simulink library "xrbsMath_r3"  (Simulink 5.0)
undefined symbols (not defined in the file or in its folder): num_width
libraries: xbsIndex_r3 x775, xrbsMath_r3 x16
(part 1 of 8)
settings Model: Creator=singhj  LastModifiedBy=singhj

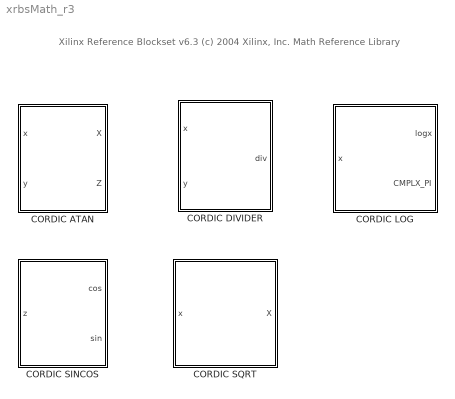
== system xrbsMath_r3 ==
  note: Xilinx Reference Blockset v6.3
      | (c) 2004  Xilinx, Inc.
      |
      | Math Reference Library
  CORDIC ATAN : Subsystem  mask{stages=8, pe_nbits=20, pe_binpt=15, pipeline_x=ones(1,8), prev_stages=8, pipeline=[1  1  1  1  1  1  1  1]}
      mask prompts: stages "Number of Processing Elements (integer value starting from 1)"; pe_nbits "X, Y Data Width"; pe_binpt "X, Y Binary Point Position"; pipeline_x "Latency for each Processing Element [1 0 0 1]"; prev_stages "Previous Number of Stages"; pipeline "Previous Pipeline Values"
      mask help: A parallel implementation, circular vectoring mode CORDIC processor for performing rectangular-to-polar conversion. The number of iteration stages (and resultant output accuracy) and the processor arithmetic precision are controlled by the mask customization.
      mask init:
      | [bg,fg] = xlcmap('XBlock',0);
      | iPos = get_param(gcb,'Position');
      | iWidth=iPos(3)-iPos(1); iHeight=iPos(4)-iPos(2);
      | iCx=iWidth/2;
      | iCy=iHeight/2;
      | [logoX, logoY] = xlogo(iPos);
      | sav_gcb=gcb;
      | stages = round(sum(abs(stages)));
      | if (stages == 0)
      | 	stages = prev_stages;
      | end
      | x = zeros(1,stages);
      | pipe_size = max(size(pipeline_x));
      | if pipe_size >= stages
      | 	x(1,1:stages) = pipeline_x(1,1:stages);
      | else
      | 	x(1,1:pipe_size) = pipeline_x(1,1:pipe_size);
      | end
      | 
      | if (stages ~=prev_stages)
      | 	pipeline=x;
      | 	cordic_pe = find_system(gcb, 'lookUnderMasks', 'all', 'FollowLinks','on','masktype', 'CORDIC parallel PE');
      |     
      |   a=find_system(cordic_pe{1}, 'lookUnderMasks', 'all', 'FollowLinks','on','masktype', 'CORDIC iteration PE');
      |   for i= 2:length(a)
      |     for j=1:3
      | 	  delete_line(cordic_pe{1}, ['CORDIC PE' int2str(i-1) '/' int2str(j)], ['CORDIC PE' int2str(i) '/' int2str(j)]);
      |     end
      |   end
      |     if length(a)>0,
      |       delete_line(cordic_pe{1}, 'x/1', 'CORDIC PE1/1');
      |       delete_line(cordic_pe{1}, 'y/1', 'CORDIC PE1/2');
      |       delete_line(cordic_pe{1}, 'z/1', 'CORDIC PE1/3');
      |       delete_line(cordic_pe{1}, ['CORDIC PE' int2str(length(a)) '/1'],'X/1');
      |       delete_line(cordic_pe{1}, ['CORDIC PE' int2str(length(a)) '/2'],'Terminator/1');
      |       delete_line(cordic_pe{1}, ['CORDIC PE' int2str(length(a)) '/3'],'Z/1');
      |     elseif length(a)==0
      |       temp_port=get_param([cordic_pe{1} '/x'],'porthandles');
      |       temp_line=get_param(temp_port.Outport,'line');
      |       if temp_line>=0  delete_line(temp_line); end
      |       temp_port=get_param([cordic_pe{1} '/y'],'porthandles');
      |       temp_line=get_param(temp_port.Outport,'line');
      |       if temp_line>=0  delete_line(temp_line); end
      |       temp_port=get_param([cordic_pe{1} '/z'],'porthandles');
      |       temp_line=get_param(temp_port.Outport,'line');
      |       if temp_line>=0  delete_line(temp_line); end
      |     end
      | 
      |     for i=2:length(a)
      |       delete_block(a{i});
      |     end
      |     for i=2:stages,
      |         add_block([cordic_pe{1} '/CORDIC PE1'], [cordic_pe{1} '/CORDIC PE' int2str(i)], 'ii', int2str(i-1),'pe_nbits', 'pe_nbits','pe_binpt', 'pe_binpt','pipeline',['pipeline(1,' int2str(i) ')'],'position',[150+(i-1)*125, 70, 205+(i-1)*125, 130]);
      |     end
      | 
      |     for i= 2:stages,
      |       for j=1:3
      | 		add_line(cordic_pe{1}, ['CORDIC PE' int2str(i-1) '/' int2str(j)], ['CORDIC PE' int2str(i) '/' int2str(j)], 'autorouting', 'on');
      |       end
      |     end
      | 
      |     if stages==0
      |       add_line(cordic_pe{1}, 'x/1', 'X/1', 'autorouting', 'on');
      |       add_line(cordic_pe{1}, 'y/1', 'Terminator/1', 'autorouting', 'on');
      |       add_line(cordic_pe{1}, 'z/1', 'Z/1', 'autorouting', 'on');
      |     elseif stages>0
      |       add_line(cordic_pe{1}, 'x/1', 'CORDIC PE1/1', 'autorouting', 'on');
      |       add_line(cordic_pe{1}, 'y/1', 'CORDIC PE1/2', 'autorouting', 'on');
      |       add_line(cordic_pe{1}, 'z/1', 'CORDIC PE1/3', 'autorouting', 'on');
      | 
      |       set_param([cordic_pe{1} '/' 'X'], 'Position', [150+stages*125, 72, 180+stages*125, 86]);
      |       set_param([cordic_pe{1} '/' 'Terminator'], 'Position', [210+stages*125, 92, 225+stages*125, 108]);
      |       set_param([cordic_pe{1} '/' 'Z'], 'Position', [240+stages*125, 113, 270+stages*125, 127]);
      | 
      |       add_line(cordic_pe{1}, ['CORDIC PE' int2str(stages) '/1'], 'X/1', 'autorouting', 'on');
      |       add_line(cordic_pe{1}, ['CORDIC PE' int2str(stages) '/2'], 'Terminator/1', 'autorouting', 'on');
      |       add_line(cordic_pe{1}, ['CORDIC PE' int2str(stages) '/3'],'Z/1', 'autorouting', 'on');
      | 
      |       % force a "compile" of the constituent constant blocks to
      |       % workaround a data propagation problem
      |       find_system(cordic_pe{1}, 'lookUnderMasks', 'all', 'FollowLinks', 'on', 'MaskType','Xilinx Constant Block');
      |   end
      | 	set_param(sav_gcb, 'prev_stages', int2str(stages));
      | 	set_param(sav_gcb, 'pipeline', [ '[' int2str(x) ']']);
      | else
      | 	if (sum(pipeline~=x))
      | 		set_param(gcb, 'pipeline', [ '[' int2str(x) ']']);
      | 	end
      | end
      | str = sprintf('-%d',sum(x) + 3);
      settings: CopyFcn=set_param(gcb, 'MaskSelfModifiable', 'on', 'LinkStatus', 'none');
      mask Help: web(xlhtmldoclink('CORDIC ATAN'));
      mask Display:
      | patch([0 iWidth iWidth 0],[0 0 iHeight iHeight] , bg);
      | patch(logoX,logoY , fg);
      | text(iCx-6,iCy,'z');
      | text(iCx,iCy+4,str);
      | port_label('input',1,'x');
      | port_label('input',2,'y');
      | port_label('output',1,'mag');
      | port_label('output',2,'atan');
      | plot([0 0 iWidth iWidth 0], [0 iHeight iHeight 0 0]);
  CORDIC DIVIDER : Subsystem  mask(CORDIC Based Divider){stages=11, num_width=16, num_binpt=11, pipeline_x=ones(1,11), prev_stages=11, pipeline=[1  1  1  1  1  1  1  1  1  1  1], prev_bits=15}
      mask prompts: stages "Number of Processing Elements (integer value starting from 1)"; num_width "X, Y, Data Width"; num_binpt "X,Y Binary Point Position"; pipeline_x "Latency for each Processing Element [1 0 0 1]"; prev_stages "Previous Number of Stages"; pipeline "Previous Pipeline Value"; prev_bits "Previous Number of Bits"
      mask help: This design implements a divider circuit using a fully parallel CORDIC (COordinate Rotation DIgital Computer) algorithm in linear vectoring mode with pre and post compensation. Using pre and post compensation techniques, this design can compute any arbitrary ratio y/x.
      mask init:
      | [bg,fg] = xlcmap('XBlock',0);
      | iPos = get_param(gcb,'Position');
      | iWidth=iPos(3)-iPos(1); iHeight=iPos(4)-iPos(2);
      | iCx=iWidth/2;
      | iCy=iHeight/2;
      | [logoX, logoY] = xlogo(iPos);
      | sav_gcb=gcb;
      | stages = round(sum(abs(stages)));
      | if (stages == 0)
      | 	stages = prev_stages;
      | end
      | x = zeros(1,stages);
      | pipe_size = max(size(pipeline_x));
      | if pipe_size >= stages
      | 	x(1,1:stages) = pipeline_x(1,1:stages);
      | else
      | 	x(1,1:pipe_size) = pipeline_x(1,1:pipe_size);
      | end
      | 
      | num_width = round(sum(abs(num_width)));
      | if (num_width < 2)
      | 	num_width = prev_bits;
      | end
      | 
      | if ((num_width-1) ~=prev_bits)
      |     % Draw the Normalization X Stage
      |     norm_x = find_system(sav_gcb, 'lookUnderMasks', 'all', 'FollowLinks','on','masktype', 'Normalize X');
      | 	a=find_system(norm_x{1}, 'lookUnderMasks', 'all', 'FollowLinks','on','masktype', 'Normalize Shift Stage');
      | 	for i= 2:length(a)
      | 		for j=1:3
      | 		    delete_line(norm_x{1}, ['Shift' int2str(i-1) '/' int2str(j)], ['Shift' int2str(i) '/' int2str(j)]);
      | 		end
      | 	end
      | 	delete_line(norm_x{1}, ['Shift' int2str(length(a)) '/1'],'norm/1');
      | 	delete_line(norm_x{1}, ['Shift' int2str(length(a)) '/2'],'shift/1');
      | 	delete_line(norm_x{1}, ['Shift' int2str(length(a)) '/3'],'Terminator1/1');
      | 	
      | 	for i=2:length(a)
      |       delete_block(a{i});
      | 	end
      | 	for i=2:(num_width-1),
      |         add_block([norm_x{1} '/Shift1'], [norm_x{1} '/Shift' int2str(i)],'position',[150+(i-1)*125, 70, 205+(i-1)*125, 130]);
      | 	end
      |     set_param([norm_x{1} '/' 'norm'], 'Position', [150+i*125, 72, 180+i*125, 86]);
      |     set_param([norm_x{1} '/' 'shift'], 'Position', [210+i*125, 92, 225+i*125, 108]);
      |     set_param([norm_x{1} '/' 'Terminator1'], 'Position', [240+i*125, 113, 270+i*125, 127]);
      |     for i= 2:(num_width-1)
      | 		for j=1:3
      | 		    add_line(norm_x{1}, ['Shift' int2str(i-1) '/' int2str(j)], ['Shift' int2str(i) '/' int2str(j)]);
      | 		end
      | 	end
      |     add_line(norm_x{1}, ['Shift' int2str((num_width-1)) '/1'],'norm/1');
      | 	add_line(norm_x{1}, ['Shift' int2str((num_width-1)) '/2'],'shift/1');
      | 	add_line(norm_x{1}, ['Shift' int2str((num_width-1)) '/3'],'Terminator1/1');
      |     
      |     % Draw the Normalization Y Stage
      |     norm_y = find_system(sav_gcb, 'lookUnderMasks', 'all', 'FollowLinks','on','masktype', 'Normalize Y');
      | 	a=find_system(norm_y{1}, 'lookUnderMasks', 'all', 'FollowLinks','on','masktype', 'Normalize Shift Stage');
      | 	for i= 2:length(a)
      | 		for j=1:3
      | 		    delete_line(norm_y{1}, ['Shift' int2str(i-1) '/' int2str(j)], ['Shift' int2str(i) '/' int2str(j)]);
      | 		end
      | 	end
      | 	delete_line(norm_y{1}, ['Shift' int2str(length(a)) '/1'],'norm/1');
      | 	delete_line(norm_y{1}, ['Shift' int2str(length(a)) '/2'],'shift/1');
      | 	delete_line(norm_y{1}, ['Shift' int2str(length(a)) '/3'],'Terminator1/1');
      | 	
      | 	for i=2:length(a)
      |       delete_block(a{i});
      | 	end
      | 	for i=2:(num_width-1)
      |         add_block([norm_y{1} '/Shift1'], [norm_y{1} '/Shift' int2str(i)],'position',[150+(i-1)*125, 70, 205+(i-1)*125, 130]);
      | 	end
      |     set_param([norm_y{1} '/' 'norm'], 'Position', [150+i*125, 72, 180+i*125, 86]);
      |     set_param([norm_y{1} '/' 'shift'], 'Position', [210+i*125, 92, 225+i*125, 108]);
      |     set_param([norm_y{1} '/' 'Terminator1'], 'Position', [240+i*125, 113, 270+i*125, 127]);
      |     for i= 2:(num_width-1)
      | 		for j=1:3
      | 		    add_line(norm_y{1}, ['Shift' int2str(i-1) '/' int2str(j)], ['Shift' int2str(i) '/' int2str(j)]);
      | 		end
      | 	end
      |     add_line(norm_y{1}, ['Shift' int2str((num_width-1)) '/1'],'norm/1');
      | 	add_line(norm_y{1}, ['Shift' int2str((num_width-1)) '/2'],'shift/1');
      | 	add_line(norm_y{1}, ['Shift' int2str((num_width-1)) '/3'],'Terminator1/1');
      | 	find_system(sav_gcb, 'lookUnderMasks', 'all', 'FollowLinks', 'on', 'MaskType','Xilinx Multiplexer Block');
      | 	set_param(sav_gcb, 'prev_bits',int2str((num_width-1)));
      | end
      | if (stages ~=prev_stages)
      | 	pipeline=x;
      |     iterative_divider = find_system(sav_gcb, 'lookUnderMasks', 'all', 'FollowLinks','on','masktype', 'CORDIC Iterative Divider');
      |   a=find_system(iterative_divider{1}, 'lookUnderMasks', 'all', 'FollowLinks','on','masktype', 'CORDIC iteration Divider');
      |   for i= 2:length(a)
      |     for j=1:3
      | 	  delete_line(iterative_divider{1}, ['CORDIC PE' int2str(i-1) '/' int2str(j)], ['CORDIC PE' int2str(i) '/' int2str(j)]);
      |     end
      |   end
      |   delete_line(iterative_divider{1}, ['CORDIC PE' int2str(length(a)) '/1'],'Terminator1/1');
      |   delete_line(iterative_divider{1}, ['CORDIC PE' int2str(length(a)) '/2'],'Terminator2/1');
      |   delete_line(iterative_divider{1}, ['CORDIC PE' int2str(length(a)) '/3'],'Z/1');
      |   for i=2:length(a)
      |      delete_block(a{i});
      |   end
      |   for i=2:stages,
      |       add_block([iterative_divider{1} '/CORDIC PE1'], [iterative_divider{1} '/CORDIC PE' int2str(i)], 'ii', int2str(i-1),'pipeline',['pipeline(1,' int2str(i) ')'],'position',[150+(i-1)*125, 70, 205+(i-1)*125, 130]);
      |   end
      |   for i= 2:stages,
      |      for j=1:3
      | 	     add_line(iterative_divider{1}, ['CORDIC PE' int2str(i-1) '/' int2str(j)], ['CORDIC PE' int2str(i) '/' int2str(j)], 'autorouting', 'on');
      |      end
      |   end
      |   set_param([iterative_divider{1} '/' 'Terminator1'], 'Position', [150+stages*125, 72, 180+stages*125, 86]);
      |   set_param([iterative_divider{1} '/' 'Terminator2'], 'Position', [210+stages*125, 92, 225+stages*125, 108]);
      |   set_param([iterative_divider{1} '/' 'Z'], 'Position', [240+stages*125, 113, 270+stages*125, 127]);
      | 
      |   add_line(iterative_divider{1}, ['CORDIC PE' int2str(stages) '/1'], 'Terminator1/1', 'autorouting', 'on');
      |   add_line(iterative_divider{1}, ['CORDIC PE' int2str(stages) '/2'], 'Terminator2/1', 'autorouting', 'on');
      |   add_line(iterative_divider{1}, ['CORDIC PE' int2str(stages) '/3'],'Z/1', 'autorouting', 'on');
      |    % force a "compile" of the constituent constant blocks to
      |    % workaround a data propagation problem
      |    find_system(iterative_divider{1}, 'lookUnderMasks', 'all', 'FollowLinks', 'on', 'MaskType','Xilinx Constant Block');
      |    set_param(sav_gcb, 'prev_stages', int2str(stages));
      |    set_param(sav_gcb, 'pipeline', [ '[' int2str(x) ']']);
      | else
      | 	if (sum(pipeline~=x))
      | 		set_param(sav_gcb, 'pipeline', [ '[' int2str(x) ']']);
      | 	end
      | end
      | 
      | str = sprintf('-%d',sum(x) + num_width + 4);
      settings: CopyFcn=set_param(gcb, 'MaskSelfModifiable', 'on', 'LinkStatus', 'none');
      mask Help: web(xlhtmldoclink('CORDIC DIVIDER'));
      mask Display:
      | patch([0 iWidth iWidth 0],[0 0 iHeight iHeight] , bg);
      | patch(logoX,logoY , fg);
      | text(iCx-6,iCy,'z');
      | text(iCx,iCy+4,str);
      | port_label('input',1,'x');
      | port_label('input',2,'y');
      | port_label('output',1,'y/x');
      | plot([0 0 iWidth iWidth 0], [0 iHeight iHeight 0 0]);
  CORDIC LOG : Subsystem  mask{stages=8, pe_nbits=8, pe_binpt=4, pipeline=ones(1,8), norm_nbits=0, norm_binpt=0}
      mask prompts: stages "Number of Processing Elements (integer value starting from 1)"; pe_nbits "Input Data Width"; pe_binpt "Input Binary Point Position"; pipeline "Latency for each Processing Element [1 0 0 1]"; norm_nbits "Normalized Data Width"; norm_binpt "Normalized Binary Point Position"
      mask help: A parallel implementation, hyperbolic vectoring mode CORDIC processor for calculating natural log of input x. The number of iteration stages (and resultant output accuracy) and the processor arithmetic precision are controlled by the mask customization.
      mask init:
      | [bg,fg] = xlcmap('XBlock',0);
      | iPos = get_param(gcb,'Position');
      | iWidth=iPos(3)-iPos(1); iHeight=iPos(4)-iPos(2);
      | iCx=iWidth/2;
      | iCy=iHeight/2;
      | [logoX, logoY] = xlogo(iPos);
      | 
      | if(length(pipeline)>stages)
      | 	x = sum(pipeline(1,1:stages));
      | else
      | 	x = sum(pipeline);
      | end
      | 
      | str = sprintf('-%d',2+pe_nbits-1+x+1);
      settings: CopyFcn=set_param(gcb, 'MaskSelfModifiable', 'on', 'LinkStatus', 'none');
      mask Help: web(xlhtmldoclink('CORDIC LOG'));
      mask Display:
      | patch([0 iWidth iWidth 0],[0 0 iHeight iHeight] , bg);
      | patch(logoX,logoY , fg);
      | text(iCx-6,iCy,'z');
      | text(iCx,iCy+4,str);
      | port_label('input',1,'x');
      | port_label('output',1,'log x');
      | port_label('output',2,'CMPLX_PI');
      | plot([0 0 iWidth iWidth 0], [0 iHeight iHeight 0 0]);
  CORDIC SINCOS : Subsystem  mask(CORDIC based Sine and Cosine function){stages=8, pe_nbits=16, pe_binpt=13, pipeline_x=ones(1,8), prev_stages=8, pipeline=[1  1  1  1  1  1  1  1]}
      mask prompts: stages "Number of Processing Elements (integer value starting from 1)"; pe_nbits "Input Data Width"; pe_binpt "Input Binary Point Position"; pipeline_x "Latency for each Processing Element [1 0 0 1]"; prev_stages "Previous Number of Stages"; pipeline "Previous Pipeline Values"
      mask help: A parallel implementation, circular rotation mode CORDIC processor for calculating Sine and Cosine of input angle z. The number of iteration stages (and resultant output accuracy) and the processor arithmetic precision are controlled by the mask customization.
      mask init:
      | [bg,fg] = xlcmap('XBlock',0);
      | iPos = get_param(gcb,'Position');
      | iWidth=iPos(3)-iPos(1); iHeight=iPos(4)-iPos(2);
      | iCx=iWidth/2;
      | iCy=iHeight/2;
      | [logoX, logoY] = xlogo(iPos);
      | sav_gcb=gcb;
      | stages = round(sum(abs(stages)));
      | if (stages == 0)
      | 	stages = prev_stages;
      | end
      | x = zeros(1,stages);
      | pipe_size = max(size(pipeline_x));
      | if pipe_size >= stages
      | 	x(1,1:stages) = pipeline_x(1,1:stages);
      | else
      | 	x(1,1:pipe_size) = pipeline_x(1,1:pipe_size);
      | end
      | 
      | if (stages ~=prev_stages)
      | 	pipeline=x;
      | 	cordic_pe = find_system(gcb, 'lookUnderMasks', 'all', 'FollowLinks','on','masktype', 'CORDIC parallel PE');
      |     
      |   a=find_system(cordic_pe{1}, 'lookUnderMasks', 'all', 'FollowLinks','on','masktype', 'CORDIC iteration PE');
      |   for i= 2:length(a)
      |     for j=1:3
      | 	  delete_line(cordic_pe{1}, ['CORDIC PE' int2str(i-1) '/' int2str(j)], ['CORDIC PE' int2str(i) '/' int2str(j)]);
      |     end
      |   end
      |     if length(a)>0,
      |       delete_line(cordic_pe{1}, 'x/1', 'CORDIC PE1/1');
      |       delete_line(cordic_pe{1}, 'y/1', 'CORDIC PE1/2');
      |       delete_line(cordic_pe{1}, 'z/1', 'CORDIC PE1/3');
      |       delete_line(cordic_pe{1}, ['CORDIC PE' int2str(length(a)) '/1'],'X/1');
      |       delete_line(cordic_pe{1}, ['CORDIC PE' int2str(length(a)) '/2'],'Y/1');
      |       delete_line(cordic_pe{1}, ['CORDIC PE' int2str(length(a)) '/3'],'Terminator/1');
      |     elseif length(a)==0
      |       temp_port=get_param([cordic_pe{1} '/x'],'porthandles');
      |       temp_line=get_param(temp_port.Outport,'line');
      |       if temp_line>=0  delete_line(temp_line); end
      |       temp_port=get_param([cordic_pe{1} '/y'],'porthandles');
      |       temp_line=get_param(temp_port.Outport,'line');
      |       if temp_line>=0  delete_line(temp_line); end
      |       temp_port=get_param([cordic_pe{1} '/z'],'porthandles');
      |       temp_line=get_param(temp_port.Outport,'line');
      |       if temp_line>=0  delete_line(temp_line); end
      |     end
      | 
      |     for i=2:length(a)
      |       delete_block(a{i});
      |     end
      |     for i=2:stages,
      |         add_block([cordic_pe{1} '/CORDIC PE1'], [cordic_pe{1} '/CORDIC PE' int2str(i)], 'ii', int2str(i-1),'pe_nbits', 'pe_nbits','pe_binpt', 'pe_binpt','pipeline',['pipeline(1,' int2str(i) ')'],'position',[150+(i-1)*125, 70, 205+(i-1)*125, 130]);
      |     end
      | 
      |     for i= 2:stages,
      |       for j=1:3
      | 		add_line(cordic_pe{1}, ['CORDIC PE' int2str(i-1) '/' int2str(j)], ['CORDIC PE' int2str(i) '/' int2str(j)], 'autorouting', 'on');
      |       end
      |     end
      | 
      |     if stages==0
      |       add_line(cordic_pe{1}, 'x/1', 'X/1', 'autorouting', 'on');
      |       add_line(cordic_pe{1}, 'y/1', 'Terminator/1', 'autorouting', 'on');
      |       add_line(cordic_pe{1}, 'z/1', 'Z/1', 'autorouting', 'on');
      |     elseif stages>0
      |       add_line(cordic_pe{1}, 'x/1', 'CORDIC PE1/1', 'autorouting', 'on');
      |       add_line(cordic_pe{1}, 'y/1', 'CORDIC PE1/2', 'autorouting', 'on');
      |       add_line(cordic_pe{1}, 'z/1', 'CORDIC PE1/3', 'autorouting', 'on');
      | 
      |       set_param([cordic_pe{1} '/' 'X'], 'Position', [150+stages*125, 72, 180+stages*125, 86]);
      |       set_param([cordic_pe{1} '/' 'Y'], 'Position', [210+stages*125, 92, 225+stages*125, 108]);
      |       set_param([cordic_pe{1} '/' 'Terminator'], 'Position', [240+stages*125, 113, 270+stages*125, 127]);
      | 
      |       add_line(cordic_pe{1}, ['CORDIC PE' int2str(stages) '/1'], 'X/1', 'autorouting', 'on');
      |       add_line(cordic_pe{1}, ['CORDIC PE' int2str(stages) '/2'], 'Y/1', 'autorouting', 'on');
      |       add_line(cordic_pe{1}, ['CORDIC PE' int2str(stages) '/3'],'Terminator/1', 'autorouting', 'on');
      | 
      |       % force a "compile" of the constituent constant blocks to
      |       % workaround a data propagation problem
      |       find_system(cordic_pe{1}, 'lookUnderMasks', 'all', 'FollowLinks', 'on', 'MaskType','Xilinx Constant Block');
      |   end
      | 	set_param(sav_gcb, 'prev_stages', int2str(stages));
      | 	set_param(sav_gcb, 'pipeline', [ '[' int2str(x) ']']);
      | else
      | 	if (sum(pipeline~=x))
      | 		set_param(gcb, 'pipeline', [ '[' int2str(x) ']']);
      | 	end
      | end
      | str = sprintf('-%d',sum(x) + 3);
      settings: CopyFcn=set_param(gcb, 'MaskSelfModifiable', 'on', 'LinkStatus', 'none');
      mask Help: web(xlhtmldoclink('CORDIC SINCOS'));
      mask Display:
      | patch([0 iWidth iWidth 0],[0 0 iHeight iHeight] , bg);
      | patch(logoX,logoY , fg);
      | text(iCx-6,iCy,'z');
      | text(iCx,iCy+4,str);
      | port_label('input',1,'z');
      | port_label('output',1,'cos');
      | port_label('output',2,'sin');
      | plot([0 0 iWidth iWidth 0], [0 iHeight iHeight 0 0]);
  CORDIC SQRT : Subsystem  mask{stages=12, pe_nbits=12, pe_binpt=6, pipeline=ones(1,12), norm_nbits=0, norm_binpt=0}
      mask prompts: stages "Number of Processing Elements (integer value starting from 1)"; pe_nbits "Input Data Width"; pe_binpt "Input Binary Point Position"; pipeline "Latency for each Processing Element [1 0 0 1]"; norm_nbits "Normalized Data Width"; norm_binpt "Normalized Binary Point"
      mask help: A parallel implementation, hyperbolic vectoring mode CORDIC processor for calculating square root of input x. The number of iteration stages (and resultant output accuracy) and the processor arithmetic precision are controlled by the mask customization.
      mask init:
      | [bg,fg] = xlcmap('XBlock',0);
      | iPos = get_param(gcb,'Position');
      | iWidth=iPos(3)-iPos(1); iHeight=iPos(4)-iPos(2);
      | iCx=iWidth/2;
      | iCy=iHeight/2;
      | [logoX, logoY] = xlogo(iPos);
      | %Normalized Data Width
      | norm_nbits = pe_binpt + (pe_nbits-pe_binpt) + mod(pe_nbits-pe_binpt-1,2);
      | norm_binpt = norm_nbits-1;
      | 
      | if(length(pipeline)>stages)
      | 	x = sum(pipeline(1,1:stages));
      | else
      | 	x = sum(pipeline);
      | end
      | 
      | str = sprintf('-%d',2+norm_binpt+1+x + 4);
      settings: CopyFcn=set_param(gcb, 'MaskSelfModifiable', 'on', 'LinkStatus', 'none');
      mask Help: web(xlhtmldoclink('CORDIC SQRT'));
      mask Display:
      | patch([0 iWidth iWidth 0],[0 0 iHeight iHeight] , bg);
      | patch(logoX,logoY , fg);
      | text(iCx-6,iCy,'z');
      | text(iCx,iCy+4,str);
      | port_label('input',1,'x');
      | port_label('output',1,'sqrt x');
      | plot([0 0 iWidth iWidth 0], [0 iHeight iHeight 0 0]);

== system xrbsMath_r3/CORDIC ATAN ==
  note: The CORDIC algorithm is implemented in 3 steps.
      |
      | Step 1: Coarse Angle Rotation.  The algorithm converges only for angles between -pi/2 and pi/2, so if x < zero, the input vector is reflected
      | to the 1st or 3rd quadrant by making the x-coordinate non-negative.
      |
      | Step 2: Fine Angle Rotation.  For rectangular-to-polar conversion, the resulting vector is rotated through progressively smaller angles, such that y goes
      | to zero. In the i-th stage, the angular rotation is by either +/- atan(1/2^i), depending on whether or not its input y is less than or greater than zero.
      |
      | Step 3: Angle Correction. If there was a reflection applied in Step 1, this step applies the appropriate angle correction by subtracting it from +/- pi.
  x : Inport
  y : Inport  Port=2
  CORDIC  Pipe Balance : xbsIndex_r3/Delay  latency=sum(pipeline)  reg_retiming=off  explicit_period=off  period=1  en=off  accept_only_valid=off  init_zero=on  dbl_ovrd=off  show_param=off
      settings: xl_area=[0, 0, 0, 0, 0, 0, 0]
  CORDIC  Pipe Balance1 : xbsIndex_r3/Delay  latency=sum(pipeline)+1  reg_retiming=off  explicit_period=off  period=1  en=off  accept_only_valid=off  init_zero=on  dbl_ovrd=off  show_param=off
      settings: xl_area=[0, 0, 0, 0, 0, 0, 0]
  CORDIC  Pipe Balance2 : xbsIndex_r3/Delay  latency=1  reg_retiming=off  explicit_period=off  period=1  en=off  accept_only_valid=off  init_zero=on  dbl_ovrd=off  show_param=off
      settings: xl_area=[0, 0, 0, 0, 0, 0, 0]
  CORDIC Fine Angle PE : Subsystem  mask(CORDIC parallel PE){}
      mask init:
      | [bg,fg] = xlcmap('XBlock',0);
      | iPos = get_param(gcb,'Position');
      | iWidth=iPos(3)-iPos(1); iHeight=iPos(4)-iPos(2);
      | iCx=iWidth/2;
      | iCy=iHeight/2;
      | [logoX, logoY] = xlogo(iPos);
      mask Display:
      | patch([0 iWidth iWidth 0],[0 0 iHeight iHeight] , bg);
      | patch(logoX,logoY , fg);
      | port_label('input',1,'x');
      | port_label('input',2,'y');
      | port_label('input',3,'z');
      | port_label('output',1,'X');
      | port_label('output',2,'Z');
      | plot([0 0 iWidth iWidth 0], [0 iHeight iHeight 0 0]);
  Constant : xbsIndex_r3/Constant  const=0  arith_type="Signed  (2's comp)"  n_bits=pe_nbits  bin_pt=pe_binpt  explicit_period=off  period=1  dbl_ovrd=off
  Quadrant Correct : Subsystem
      mask init:
      | [bg,fg] = xlcmap('XBlock',0);
      | iPos = get_param(gcb,'Position');
      | iWidth=iPos(3)-iPos(1); iHeight=iPos(4)-iPos(2);
      | iCx=iWidth/2;
      | iCy=iHeight/2;
      | [logoX, logoY] = xlogo(iPos);
      mask Display:
      | patch([0 iWidth iWidth 0],[0 0 iHeight iHeight] , bg);
      | patch(logoX,logoY , fg);
      | port_label('input',1,'Z in');
      | port_label('input',2,'sgn(y)');
      | port_label('input',3,'sgn(x)');
      | port_label('output',1,'Z');
      | plot([0 0 iWidth iWidth 0], [0 iHeight iHeight 0 0]);
  Quadrant Map : Subsystem
      mask init:
      | [bg,fg] = xlcmap('XBlock',0);
      | iPos = get_param(gcb,'Position');
      | iWidth=iPos(3)-iPos(1); iHeight=iPos(4)-iPos(2);
      | iCx=iWidth/2;
      | iCy=iHeight/2;
      | [logoX, logoY] = xlogo(iPos);
      mask Display:
      | patch([0 iWidth iWidth 0],[0 0 iHeight iHeight] , bg);
      | patch(logoX,logoY , fg);
      | port_label('input',1,'x');
      | port_label('input',2,'y');
      | port_label('output',1,'X');
      | port_label('output',2,'Y');
      | port_label('output',3,'sgn(y)');
      | port_label('output',4,'sgn(x)');
      | plot([0 0 iWidth iWidth 0], [0 iHeight iHeight 0 0]);
  X : Outport
  Z : Outport  Port=2
  wires:
  CORDIC  Pipe Balance2/1 -> X/1
  CORDIC Fine Angle PE/1(X) -> CORDIC  Pipe Balance2/1
  Quadrant Correct/1(Z) -> Z/1
  CORDIC Fine Angle PE/2(Z) -> Quadrant Correct/1(Z IN)
  CORDIC  Pipe Balance1/1 -> Quadrant Correct/3(Z MUX SEL)
  CORDIC  Pipe Balance/1 -> Quadrant Correct/2(PI_ addsub)
  Quadrant Map/4(sign(x)) -> CORDIC  Pipe Balance1/1
  Quadrant Map/3(sign(y)) -> CORDIC  Pipe Balance/1
  y/1 -> Quadrant Map/2(y)
  x/1 -> Quadrant Map/1(x)
  Quadrant Map/2(Y) -> CORDIC Fine Angle PE/2(y)
  Quadrant Map/1(X) -> CORDIC Fine Angle PE/1(x)
  Constant/1 -> CORDIC Fine Angle PE/3(z)

== system xrbsMath_r3/CORDIC DIVIDER ==
  note: The CORDIC Divider algorithm is implemented in 4 steps.
      |
      | Step 1: Co-ordinate Rotation.  The CORDIC algorithm converges only for positive values of x, so if x < zero, the input vector is
      | reflected to the 1st or 3rd quadrant by making the x-coordinate non-negative. For normalizing X and Y, Y is always mapped to
      | a non-negative value. The Divider circuit has been designed to converge for all values of X and Y, except for the most negative value .
      |
      | Step 2: Normalization.  The CORDIC algorithm converges only for y <= 2 x. For  x > y, both the inputs X and Y are shifted to the
      | left till they have a 1 in the most significant bit (MSB).  The relative shift of Y over X is recorded and passed on to the Quadrant
      | Correct Stage.
      |
      | Step 3: Linear Rotations.  For ratio calculation, the resulting vector is rotated through progressively smaller angles, such that y goes
      | to zero. In the i-th stage, the rotation yields +/- y/x, depending on whether the input y is less than or greater than zero.
      |
      | Step 4: Co-ordinate Correction. If the axis was rotated Step 1 and a relative shift was applied to Y over X, this step assigns the appropriate
      | sign to the resulting ratio and multiplies it with 2^(relative_shift of Y over X).
  x : Inport
  y : Inport  Port=2
  Constant2 : xbsIndex_r3/Constant  const=0  arith_type="Signed  (2's comp)"  n_bits=stages+2  bin_pt=stages  explicit_period=off  period=1  dbl_ovrd=off
  Delay : xbsIndex_r3/Delay  latency=sum(pipeline)  reg_retiming=off  explicit_period=off  period=1  en=off  accept_only_valid=off  init_zero=on  dbl_ovrd=off
      settings: xl_area=[1 1 0 1 0 0 0]
  Delay1 : xbsIndex_r3/Delay  latency=sum(pipeline)  reg_retiming=off  explicit_period=off  period=1  en=off  accept_only_valid=off  init_zero=on  dbl_ovrd=off
      settings: xl_area=[2 4 0 4 0 0 0]
  Iterative Divider : Subsystem  mask(CORDIC Iterative Divider){}
      mask init:
      | [bg,fg] = xlcmap('XBlock',0);
      | iPos = get_param(gcb,'Position');
      | iWidth=iPos(3)-iPos(1); iHeight=iPos(4)-iPos(2);
      | iCx=iWidth/2;
      | iCy=iHeight/2;
      | [logoX, logoY] = xlogo(iPos);
      mask Display:
      | patch([0 iWidth iWidth 0],[0 0 iHeight iHeight] , bg);
      | patch(logoX,logoY , fg);
      | port_label('input',1,'x');
      | port_label('input',2,'y');
      | port_label('input',3,'z');
      | port_label('output',1,'Z');
      | plot([0 0 iWidth iWidth 0], [0 iHeight iHeight 0 0]);
  Quadrant Correct : Subsystem  mask{num_width=num_width, num_binpt=num_binpt}
      mask prompts: num_width "Data Width"; num_binpt "Data Binary Point"
      mask init:
      | [bg,fg] = xlcmap('XBlock',0);
      | iPos = get_param(gcb,'Position');
      | iWidth=iPos(3)-iPos(1); iHeight=iPos(4)-iPos(2);
      | iCx=iWidth/2;
      | iCy=iHeight/2;
      | [logoX, logoY] = xlogo(iPos);
      mask Display:
      | patch([0 iWidth iWidth 0],[0 0 iHeight iHeight] , bg);
      | patch(logoX,logoY , fg);
      | port_label('input',1,'z');
      | port_label('input',2,'sign');
      | port_label('input',3,'norm');
      | port_label('output',1,'y/x');
      | plot([0 0 iWidth iWidth 0], [0 iHeight iHeight 0 0]);
  Quadrant Map : Subsystem  mask{num_width=num_width, num_binpt=num_binpt}
      mask prompts: num_binpt "Num_bin_pt"
      mask init:
      | [bg,fg] = xlcmap('XBlock',0);
      | iPos = get_param(gcb,'Position');
      | iWidth=iPos(3)-iPos(1); iHeight=iPos(4)-iPos(2);
      | iCx=iWidth/2;
      | iCy=iHeight/2;
      | [logoX, logoY] = xlogo(iPos);
      mask Display:
      | patch([0 iWidth iWidth 0],[0 0 iHeight iHeight] , bg);
      | patch(logoX,logoY , fg);
      | port_label('input',1,'x');
      | port_label('input',2,'y');
      | port_label('output',1,'norm_x');
      | port_label('output',2,'norm_y');
      | port_label('output',3,'sign');
      | port_label('output',4,'index');
      | plot([0 0 iWidth iWidth 0], [0 iHeight iHeight 0 0]);
  div : Outport
  wires:
  Constant2/1 -> Iterative Divider/3(z)
  Quadrant Map/1(norm_X) -> Iterative Divider/1(x)
  Quadrant Map/2(norm_Y) -> Iterative Divider/2(y)
  Iterative Divider/1(Z) -> Quadrant Correct/1(z)
  Quadrant Map/3(sign) -> Delay/1
  Delay/1 -> Quadrant Correct/2(sign)
  Quadrant Map/4(index) -> Delay1/1
  Delay1/1 -> Quadrant Correct/3(norm)
  x/1 -> Quadrant Map/1(x)
  y/1 -> Quadrant Map/2(y)
  Quadrant Correct/1(Z) -> div/1

== system xrbsMath_r3/CORDIC LOG ==
  note: The CORDIC Natural Log algorithm is implemented in 4 steps.
      |
      | Step 1: Co-ordinate Rotation.  The CORDIC algorithm converges only for positive values of x. If x < zero, the input data is
      | converted to a non-negative number. If x = 0, a zero detect flag is passed along to the output stage. The Log circuit has been
      | designed to converge for all values of X, except for the most negative value .
      |
      | Step 2: Normalization.  The CORDIC algorithm converges only for 0.5 <= x < 1.0. During normalization, the input X is shifted to the
      | left till it has a 1 in the most significant bit.The log output is derived using the identity log( w) = 2*atanh{ (w-l) / (w+1) }.
      | Based on this identity the input w gets mapped to, X = w + 1 and Y = w - 1.
      |
      | Step 3: Hyperbolic Rotations.  For atanh{ (w-l) / (w+1) }. calculation, the resulting vector is rotated through progressively smaller
      | angles, such that y goes to zero.
      |
      | Step 4: Co-ordinate Correction. If the input was negative  a CMPLX_PI flag is porvided at the output for adding PI if a complex output is desired.
      | If a left shift was applied to X, this step adjusts the output by using the equation log (w * 2^E) = log (w) + E * log (2).
  x : Inport
  CORDIC Fine Angle PE : Subsystem  mask(CORDIC parallel PE){stages=stages, pe_nbits=pe_nbits+1, pe_binpt=pe_nbits-1, pipeline_x=pipeline, prev_stages=8, pipeline=[1  1  1  1  1  1  1  1]}
      mask prompts: stages "Number of Stages"; pe_nbits "Number of Bits"; pe_binpt "Binary Point Position"; pipeline_x "Pipeline Stage Value"; prev_stages "Previous Stages"; pipeline "Previous Pipeline Stage Value"
      mask init:
      | [bg,fg] = xlcmap('XBlock',0);
      | iPos = get_param(gcb,'Position');
      | iWidth=iPos(3)-iPos(1); iHeight=iPos(4)-iPos(2);
      | iCx=iWidth/2;
      | iCy=iHeight/2;
      | [logoX, logoY] = xlogo(iPos);
      | set_param(gcb,'LinkStatus', 'none');
      | sav_gcb=gcb;
      | stages = round(sum(abs(stages)));
      | if (stages == 0)
      | 	stages = prev_stages;
      | end
      | x = zeros(1,stages);
      | pipe_size = max(size(pipeline_x));
      | if pipe_size >= stages
      | 	x(1,1:stages) = pipeline_x(1,1:stages);
      | else
      | 	x(1,1:pipe_size) = pipeline_x(1,1:pipe_size);
      | end
      | 
      | if (stages ~=prev_stages)
      | 	pipeline = x;
      | 	a=find_system(sav_gcb, 'lookUnderMasks', 'all', 'FollowLinks','on','masktype', 'CORDIC iteration PE');
      | 	for i= 2:length(a)
      | 		for j=1:3
      | 		    delete_line(sav_gcb, ['CORDIC PE' int2str(i-1) '/' int2str(j)], ['CORDIC PE' int2str(i) '/' int2str(j)]);
      | 		end
      | 	end
      | 	delete_line(sav_gcb, ['CORDIC PE' int2str(length(a)) '/1'],'T1/1');
      | 	delete_line(sav_gcb, ['CORDIC PE' int2str(length(a)) '/2'],'T2/1');
      | 	delete_line(sav_gcb, ['CORDIC PE' int2str(length(a)) '/3'],'Z/1');
      | 	
      | 	for i=2:length(a)
      |       delete_block(a{i});
      | 	end
      | 	ite_stage=1;
      | 	repeat_stage=4;
      | 	dec_stage=0;
      | 	for i=2:stages
      |         ite_stage= i-dec_stage;
      | 		if(repeat_stage==ite_stage-1)
      |             ite_stage=ite_stage-1;
      | 			repeat_stage=repeat_stage*3+1;
      | 			dec_stage=dec_stage+1;
      | 		end
      |         add_block([sav_gcb '/CORDIC PE1'], [sav_gcb '/CORDIC PE' int2str(i)],'ii',int2str(ite_stage),'pipeline',['pipeline(1,' int2str(i) ')'],'position',[150+(i-1)*125, 70, 205+(i-1)*125, 130]);
      | 	end
      |     set_param([sav_gcb '/' 'T1'], 'Position', [150+stages*125, 73, 180+stages*125, 87]);
      |     set_param([sav_gcb '/' 'T2'], 'Position', [210+stages*125, 92, 225+stages*125, 108]);
      | 	set_param([sav_gcb '/' 'Z'], 'Position', [270+stages*125, 111, 270+stages*125, 129]);
      |     for i= 2:stages
      | 		for j=1:3
      | 		    add_line(sav_gcb, ['CORDIC PE' int2str(i-1) '/' int2str(j)], ['CORDIC PE' int2str(i) '/' int2str(j)]);
      | 		end
      | 	end
      |     add_line(sav_gcb, ['CORDIC PE' int2str(stages) '/1'],'T1/1');
      | 	add_line(sav_gcb, ['CORDIC PE' int2str(stages) '/2'],'T2/1');
      | 	add_line(sav_gcb, ['CORDIC PE' int2str(stages) '/3'],'Z/1');
      | 	find_system(sav_gcb, 'lookUnderMasks', 'all', 'FollowLinks', 'on', 'MaskType','Xilinx Slice Block');
      | 	set_param(sav_gcb, 'prev_stages',int2str(stages));
      | 	set_param(sav_gcb, 'pipeline', [ '[' int2str(x) ']']);
      | end
      | 
      | if (sum(pipeline~=x))
      | 	pipeline = x;
      | 	set_param(sav_gcb, 'pipeline', [ '[' int2str(x) ']']);
      | end
      mask Display:
      | patch([0 iWidth iWidth 0],[0 0 iHeight iHeight] , bg);
      | patch(logoX,logoY , fg);
      | port_label('input',1,'x');
      | port_label('input',2,'y');
      | port_label('input',3,'z');
      | port_label('input',4,'shift');
      | port_label('input',5,'sgn(x)');
      | port_label('input',6,'0_det');
      | port_label('output',1,'Z');
      | port_label('output',2,'shift');
      | port_label('output',3,'sgn(x)');
      | port_label('output',4,'0_det');
      | plot([0 0 iWidth iWidth 0], [0 iHeight iHeight 0 0]);
  Quadrant Correct : Subsystem  mask{pe_nbits=pe_nbits, pe_binpt=pe_binpt, k_val=0, k_bits=0}
      mask prompts: pe_nbits "Number of Bits"; pe_binpt "Binary Point Position"; k_val "Constant Value"; k_bits "Constant Bits"
      mask init:
      | [bg,fg] = xlcmap('XBlock',0);
      | iPos = get_param(gcb,'Position');
      | iWidth=iPos(3)-iPos(1); iHeight=iPos(4)-iPos(2);
      | iCx=iWidth/2;
      | iCy=iHeight/2;
      | [logoX, logoY] = xlogo(iPos);
      | t = pe_nbits-pe_binpt-1;
      | if (t== 0)
      | 	k_val = 0;
      | 	k_bits = 1;
      | else
      | 	k_val= t;
      | 	k_bits = ceil(log2(t+1));
      | end
      mask Display:
      | patch([0 iWidth iWidth 0],[0 0 iHeight iHeight] , bg);
      | patch(logoX,logoY , fg);
      | port_label('input',1,'X');
      | port_label('input',2,'shift');
      | port_label('input',3,'sgn(x)');
      | port_label('input',4,'0_det');
      | port_label('output',1,'log X');
      | port_label('output',2,'CMPLX_PI');
      | plot([0 0 iWidth iWidth 0], [0 iHeight iHeight 0 0]);
  Quadrant Map : Subsystem
      mask init:
      | [bg,fg] = xlcmap('XBlock',0);
      | iPos = get_param(gcb,'Position');
      | iWidth=iPos(3)-iPos(1); iHeight=iPos(4)-iPos(2);
      | iCx=iWidth/2;
      | iCy=iHeight/2;
      | [logoX, logoY] = xlogo(iPos);
      mask Display:
      | patch([0 iWidth iWidth 0],[0 0 iHeight iHeight] , bg);
      | patch(logoX,logoY , fg);
      | port_label('input',1,'x');
      | port_label('output',1,'X');
      | port_label('output',2,'Y');
      | port_label('output',3,'Z');
      | port_label('output',4,'shift');
      | port_label('output',5,'sgn(x)');
      | port_label('output',6,'0_det');
      | plot([0 0 iWidth iWidth 0], [0 iHeight iHeight 0 0]);
  logx : Outport
  CMPLX_PI : Outport  Port=2
  wires:
  CORDIC Fine Angle PE/3(sign_dly) -> Quadrant Correct/3(sign_x)
  CORDIC Fine Angle PE/2(shift_dly) -> Quadrant Correct/2(shift)
  Quadrant Map/5(sign) -> CORDIC Fine Angle PE/5(sign)
  Quadrant Map/6(zero_detect) -> CORDIC Fine Angle PE/6(zero_detect)
  Quadrant Map/4(shift1) -> CORDIC Fine Angle PE/4(shift1)
  Quadrant Map/3(shift) -> CORDIC Fine Angle PE/3(z)
  Quadrant Map/2(Y) -> CORDIC Fine Angle PE/2(y)
  Quadrant Map/1(X) -> CORDIC Fine Angle PE/1(x)
  Quadrant Correct/2(CMPLX_PI) -> CMPLX_PI/1
  CORDIC Fine Angle PE/4(zero_detect_dly) -> Quadrant Correct/4(zero_detect)
  x/1 -> Quadrant Map/1(x)
  CORDIC Fine Angle PE/1(Z) -> Quadrant Correct/1(X)
  Quadrant Correct/1(Z) -> logx/1

== system xrbsMath_r3/CORDIC SINCOS ==
  note: The CORDIC algorithm is implemented in 3 steps.
      |
      | Step 1: Coarse Angle Rotation.  The algorithm converges only for angles between -pi/2 and pi/2. If  z > pi/2, the input angle is reflected
      |  to the 1st quadrant by subtracting pi/2 from the input angle. When z < -pi/2, the input angle is reflected back to the 3rd quadrant by adding
      | pi/2 to the input angle .
      |
      | Step 2: Fine Angle Rotation.  By setting x equal to 1/1.646760 and y equal to 0, the rotational mode CORDIC processor yields cosine and sine
      | of the input angle Z.
      |
      | Step 3: Angle Correction. If there was a reflection applied in Step 1, this step applies the appropriate correction .
  z : Inport
  CORDIC Fine Angle PE : Subsystem  mask(CORDIC parallel PE){}
      mask init:
      | [bg,fg] = xlcmap('XBlock',0);
      | iPos = get_param(gcb,'Position');
      | iWidth=iPos(3)-iPos(1); iHeight=iPos(4)-iPos(2);
      | iCx=iWidth/2;
      | iCy=iHeight/2;
      | [logoX, logoY] = xlogo(iPos);
      mask Display:
      | patch([0 iWidth iWidth 0],[0 0 iHeight iHeight] , bg);
      | patch(logoX,logoY , fg);
      | port_label('input',1,'x');
      | port_label('input',2,'y');
      | port_label('input',3,'z');
      | port_label('output',1,'X');
      | port_label('output',2,'Y');
      | plot([0 0 iWidth iWidth 0], [0 iHeight iHeight 0 0]);
  Constant : xbsIndex_r3/Constant  const=1/1.646760  arith_type="Signed  (2's comp)"  n_bits=pe_nbits  bin_pt=pe_binpt  explicit_period=off  period=1  dbl_ovrd=off
  Constant1 : xbsIndex_r3/Constant  const=0  arith_type="Signed  (2's comp)"  n_bits=pe_nbits  bin_pt=pe_binpt  explicit_period=off  period=1  dbl_ovrd=off
  Delay1 : xbsIndex_r3/Delay  latency=sum(pipeline)+2  reg_retiming=off  explicit_period=off  period=1  en=off  accept_only_valid=off  init_zero=on  dbl_ovrd=off  show_param=off
      settings: xl_area=[1 1 0 1 0 0 0]
  Delay4 : xbsIndex_r3/Delay  latency=sum(pipeline)+1  reg_retiming=off  explicit_period=off  period=1  en=off  accept_only_valid=off  init_zero=on  dbl_ovrd=off  show_param=off
      settings: xl_area=[1 1 0 1 0 0 0]
  Quadrant Correct : Subsystem
      mask init:
      | [bg,fg] = xlcmap('XBlock',0);
      | iPos = get_param(gcb,'Position');
      | iWidth=iPos(3)-iPos(1); iHeight=iPos(4)-iPos(2);
      | iCx=iWidth/2;
      | iCy=iHeight/2;
      | [logoX, logoY] = xlogo(iPos);
      mask Display:
      | patch([0 iWidth iWidth 0],[0 0 iHeight iHeight] , bg);
      | patch(logoX,logoY , fg);
      | port_label('input',1,'x');
      | port_label('input',2,'y');
      | port_label('input',3,'angle_map');
      | port_label('input',4,'sgn(z)');
      | port_label('output',1,'cos');
      | port_label('output',2,'sin');
      | plot([0 0 iWidth iWidth 0], [0 iHeight iHeight 0 0]);
  Quadrant Map : Subsystem
      mask init:
      | [bg,fg] = xlcmap('XBlock',0);
      | iPos = get_param(gcb,'Position');
      | iWidth=iPos(3)-iPos(1); iHeight=iPos(4)-iPos(2);
      | iCx=iWidth/2;
      | iCy=iHeight/2;
      | [logoX, logoY] = xlogo(iPos);
      mask Display:
      | patch([0 iWidth iWidth 0],[0 0 iHeight iHeight] , bg);
      | patch(logoX,logoY , fg);
      | port_label('input',1,'z');
      | port_label('output',1,'z');
      | port_label('output',2,'angle_map');
      | port_label('output',3,'sgn(z)');
      | plot([0 0 iWidth iWidth 0], [0 iHeight iHeight 0 0]);
  cos : Outport
  sin : Outport  Port=2
  wires:
  Quadrant Correct/1(cosine) -> cos/1
  Quadrant Correct/2(sine) -> sin/1
  Constant1/1 -> CORDIC Fine Angle PE/2(y)
  Constant/1 -> CORDIC Fine Angle PE/1(x)
  Quadrant Map/1(Z) -> CORDIC Fine Angle PE/3(z)
  Quadrant Map/3(sgn_z) -> Delay1/1
  Quadrant Map/2(angle_map) -> Delay4/1
  z/1 -> Quadrant Map/1(z)
  Delay4/1 -> Quadrant Correct/3(angle_map)
  Delay1/1 -> Quadrant Correct/4(sgn(z))
  CORDIC Fine Angle PE/2(Y) -> Quadrant Correct/2(sin)
  CORDIC Fine Angle PE/1(X) -> Quadrant Correct/1(cos)
